simulink model "full_wave2"  (R2019a)
settings: Solver=VariableStepAuto  StartTime=0.0  StopTime=10.0  RelTol=1e-3
libraries: powerlib x9
settings Model: ModifiedByFormat=Yasir Jabbar  Creator=Yasir Jabbar  LastModifiedBy=Yasir Jabbar

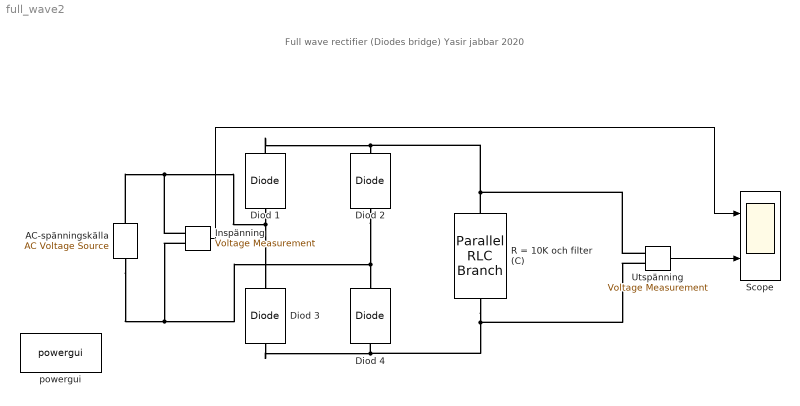
== system full_wave2 ==
  note: Full wave rectifier
      | (Diodes bridge)
      | Yasir jabbar
      | 2020
  AC-spänningskälla : powerlib/Electrical Sources/AC Voltage Source  Amplitude=12  Phase=0  Frequency=60  SampleTime=0  Measurements=None  BusType=swing  Pref=10e3  Qref=0  Qmin=-inf  Qmax=+inf
      settings: SourceProductName=Simscape Electrical
  Diod {1..4} (4 alike) : powerlib/Power Electronics/Diode  Ron=0.001  Lon=0  Vf=0.7  IC=0  UseSnubber=off  Rs=500  Cs=inf  Measurements=off
      settings: SourceProductName=Simscape Electrical
  "Inspänning " : powerlib/Measurements/Voltage Measurement  PhasorSimulation=off  OutputType=Complex  PSBequivalent=0
  R = 10K och filter (C) : powerlib/Elements/Parallel RLC Branch  LConnTagsString=a  RConnTagsString=__new0  BranchType=RC  Resistance=10000  Inductance=1e-3  SetiL0=off  InitialCurrent=0  Capacitance=100e-6  Setx0=off  InitialVoltage=0  Measurements=None
  Scope : Scope  NumInputPorts=2
  Utspänning : powerlib/Measurements/Voltage Measurement  PhasorSimulation=off  OutputType=Complex  PSBequivalent=0
  powergui : powerlib/powergui  Priority=1  SimulationMode=Discrete  SampleTime=50e-6  frequency=60  Iterations=50  frequencyindice=0  Pbase=100e6  ErrMax=1e-4  UnitsV=kV  UnitsW=MW  buscounter=0  FunctionMessages=off  echomessages=off  EnableUseOfTLC=off  CurrentSourceSwitches=off  DisableSnubberDevices=off  DisableRonSwitches=off  DisableVfSwitches=off  DisplayEquations=off  AutomaticDiscreteSolvers=off  SolverType=Tustin/Backward Euler (TBE)  Interpol=off  ExternalGateDelay=off  methode=off  Ts=100  x0status=blocks  SPID=on  SwTol=0  HookPort=off  NonlinearTolerance=0  nMaxIteration=15  ContinueOnMaxIteration=off  RestoreLinks=warning  ResistiveCurrentMeasurement=off  Frange=[0:2:500]  Ylog=off  Xlog=on  ShowGrid=off  save=off  variable=ZData  structure=0  ZoomFFT=off  StartTime=0.0  cycles=1  DisplayStyle=1  fundamental=60  FreqAxis=off  MaxFrequency=1000  frequencyindicesteady=1  RmsSteady=1  display=off
      settings: SourceProductName=Simscape Electrical
  wires:
  "Inspänning "/1 -> Scope/1
  Utspänning/1 -> Scope/2
  connections:
  Diod 1/LConn1 -- "Inspänning "/LConn1 -- AC-spänningskälla/RConn1 -- Diod 3/RConn1
  Diod 2/LConn1 -- "Inspänning "/LConn2 -- AC-spänningskälla/LConn1 -- Diod 4/RConn1
  Diod 1/RConn1 -- Utspänning/LConn1 -- R = 10K och filter (C)/RConn1 -- Diod 2/RConn1
  Diod 3/LConn1 -- R = 10K och filter (C)/LConn1 -- Utspänning/LConn2 -- Diod 4/LConn1
